simulink model "clearing_faulted_segment_travelling_Wave"  (R2018a)
settings: Solver=ode23t  StartTime=0.0  StopTime=2  MaxStep=1e-3  RelTol=1e-3
values from neighbouring files (symbols this model uses):
  AC_lim = [1.5 -1.5]    [MT_HVDC_initialize.m]
  C_pm = 10.48e-3    (= 0.01048)    [MT_HVDC_initialize.m]
  ccsc_lim = [1.0 -1.0]    [MT_HVDC_initialize.m]
  DC_lim = [1.05 -1.05]    [MT_HVDC_initialize.m]
  f = 50    [MT_HVDC_initialize.m]
  Fc = 50    [MT_HVDC_initialize.m]
  Fn_filter = 1000    [MT_HVDC_initialize.m]
  Ireg_lim_i = [1.5, -1.5]    [MT_HVDC_initialize.m]
  Ireg_lim_r = [1.5, -1.5]    [MT_HVDC_initialize.m]
  Ki_ACreg_i = 260    [MT_HVDC_initialize.m]
  Ki_ccsc = 5    [MT_HVDC_initialize.m]
  Ki_DCreg_r = 150    [MT_HVDC_initialize.m]
  Ki_Ireg_i = 200    [MT_HVDC_initialize.m]
  Ki_Ireg_r = 100    [MT_HVDC_initialize.m]
  Ki_R_inv = 150000    [MT_HVDC_initialize.m]
  Ki_R_rec = 5000    [MT_HVDC_initialize.m]
  Kp_ACreg_i = 2    [MT_HVDC_initialize.m]
  Kp_ccsc = 1    [MT_HVDC_initialize.m]
  Kp_DCreg_r = 8    [MT_HVDC_initialize.m]
  Kp_Ireg_i = 2    [MT_HVDC_initialize.m]
  Kp_Ireg_r = 2    [MT_HVDC_initialize.m]
  Kp_R_inv = 0.001    [MT_HVDC_initialize.m]
  Kp_R_rec = 0.001    [MT_HVDC_initialize.m]
  L1_pu = 0.109    [MT_HVDC_initialize.m]
  L2_pu = 0.0824    [MT_HVDC_initialize.m]
  L_arm = L_arm_pu*Z_base66/w    [MT_HVDC_initialize.m]
  L_arm_pu = 0.15    [MT_HVDC_initialize.m]
  L_int = X_int/w    [MT_HVDC_initialize.m]
  n = 50    [MT_HVDC_initialize.m]
  n2 = 50    [MT_HVDC_initialize.m]
  P_nom = 220e6    (= 220000000)    [MT_HVDC_initialize.m]
  R1_pu = 0.00206    [MT_HVDC_initialize.m]
  R2_pu = 0.00206    [MT_HVDC_initialize.m]
  R_arm = 0.03    [MT_HVDC_initialize.m]
  R_arm_pu = R_arm/Z_base66    [MT_HVDC_initialize.m]
  R_int = sqrt((z_int_400^2)/(1+xr_ratio^2))    [MT_HVDC_initialize.m]
  Rg_T1 = 40    [MT_HVDC_initialize.m]
  S1_nom = P_nom    (= 220000000)    [MT_HVDC_initialize.m]
  S2_nom = P_nom    (= 220000000)    [MT_HVDC_initialize.m]
  T_fault = 1.4    [MT_HVDC_initialize.m]
  Ts_Control = 40e-6    (= 4e-05)    [MT_HVDC_initialize.m]
  Ts_Power = 20e-6    (= 2e-05)    [MT_HVDC_initialize.m]
  V1_prim = V_prim    (= 400000)    [MT_HVDC_initialize.m]
  V1_sec = V_grid    (= 66000)    [MT_HVDC_initialize.m]
  V2_prim = V_grid    (= 66000)    [MT_HVDC_initialize.m]
  V2_sec = 18e3    (= 18000)    [MT_HVDC_initialize.m]
  V_ac_ref = 1.035    [MT_HVDC_initialize.m]
  V_grid = 66e3    (= 66000)    [MT_HVDC_initialize.m]
  V_prim = 400e3    (= 400000)    [MT_HVDC_initialize.m]
  Vc_pm_r = 0*Vdc_nom/n    (= 0)    [MT_HVDC_initialize.m]
  Vdc_nom = 135e3    (= 135000)    [MT_HVDC_initialize.m]
  w = 2*pi*f    (= 314.159265359)    [MT_HVDC_initialize.m]
  z0z1 = 0.8    [MT_HVDC_initialize.m]
  Zeta_filter = 1    [MT_HVDC_initialize.m]
undefined symbols (not defined in the file or in its folder): D1, Delta, DiscIntNeverNeededParam
libraries: powerlib x417, powerlib_meascontrol x130, simulink x84, powerlib_extras x8, simulink_extras x5
(part 14 of 17)

== system clearing_faulted_segment_travelling_Wave/MMC Converter2/Half-Bridge MMC Ap2/HalfBridgeMMC_Agt_Discrete ==
  N : Inport  PortDimensions=2
  Current Measurement1 : powerlib/Measurements/Current Measurement  PhasorSimulation=off  OutputType=Complex  PSBequivalent=0
      settings: SourceProductName=Simscape Electrical
  Current Measurement2 : powerlib/Measurements/Current Measurement  PhasorSimulation=off  OutputType=Complex  PSBequivalent=0
      settings: SourceProductName=Simscape Electrical
  Demux : Demux  Outputs=2
  Discrete-Time Integrator : DiscreteIntegrator  IntegratorMethod=Integration: Trapezoidal  gainval=1  InitialCondition=Vc_Initial  SampleTime=Ts  UpperSaturationLimit=5000  LowerSaturationLimit=500  ICPrevOutput=DiscIntNeverNeededParam  ICPrevScaledInput=DiscIntNeverNeededParam
  Dp : powerlib/Power Electronics/Diode  Ron=Ron_Diode  Lon=0  Vf=Vf_Diode  IC=0  UseSnubber=off  Rs=Rs_Diode  Cs=Cs_Diode  Measurements=off
      settings: SourceProductName=Simscape Electrical
  Dp2 : powerlib/Power Electronics/Diode  Ron=Ron_Diode  Lon=0  Vf=Vf_Diode  IC=0  UseSnubber=off  Rs=Rs_Diode  Cs=Cs_Diode  Measurements=off
      settings: SourceProductName=Simscape Electrical
  Gain : Gain  Gain=1/(C*n)
  Gain2 : Gain  Gain=2
  Mux : Mux  Inputs=2
  Product1 : Product
  Product2 : Product
  Saturation1 : Saturate  UpperLimit=n  LowerLimit=0
  Sum1 : Sum  Inputs=1  SaturateOnIntegerOverflow=on  InputSameDT=on  OutDataTypeStr=Inherit: Same as first input
  Sum2 : Sum  Inputs=+-  SaturateOnIntegerOverflow=on  InputSameDT=on  OutDataTypeStr=Inherit: Same as first input
  Unit Delay1 : UnitDelay  SampleTime=Ts
  Unit Delay3 : UnitDelay  InitialCondition=Vc_Initial  SampleTime=Ts
  Unit Delay4 : UnitDelay  InitialCondition=Vc_Initial  SampleTime=Ts
  Vp : powerlib/Electrical Sources/Controlled Voltage Source  Initialize=off  Source_Type=AC  Amplitude=0  Phase=0  Frequency=0  Measurements=None
      settings: SourceProductName=Simscape Electrical
  Vp1 : powerlib/Electrical Sources/Controlled Voltage Source  Initialize=off  Source_Type=AC  Amplitude=0  Phase=0  Frequency=0  Measurements=None
      settings: SourceProductName=Simscape Electrical
  1 : PMIOPort  Side=Left
  2 : PMIOPort  Port=2  Side=Left
  Vc : Outport
  wires:
  Sum1/1 -> Gain/1
  Sum2/1 -> Vc/1, Product2/2
  Product1/1 -> Sum1/1
  Saturation1/1 -> Product2/1, Product1/1
  Unit Delay1/1 -> Product1/2
  [Icap] -> Mux/2
  [Vbl] -> Vp1/1
  Current Measurement2/1 -> [Icap]
  Current Measurement1/1 -> [Imod]
  [Vin] -> Vp/1
  Demux/2 -> [Vbl]
  Demux/1 -> [Vin]
  Product2/1 -> Demux/1
  Mux/1 -> Unit Delay1/1
  Discrete-Time Integrator/1 -> Unit Delay4/1
  Gain/1 -> Discrete-Time Integrator/1
  Gain2/1 -> Sum2/1
  Unit Delay4/1 -> Gain2/1, Unit Delay3/1
  Unit Delay3/1 -> Sum2/2
  [Imod] -> Mux/1
  N/1 -> Saturation1/1
  connections:
  Dp2/LConn1 -- 2/RConn1 -- Vp1/LConn1
  Vp1/RConn1 -- Current Measurement2/RConn1
  Current Measurement2/LConn1 -- Dp/RConn1
  Dp2/RConn1 -- Dp/LConn1 -- Current Measurement1/RConn1
  Vp/LConn1 -- Current Measurement1/LConn1
  1/RConn1 -- Vp/RConn1

== system clearing_faulted_segment_travelling_Wave/MMC Converter2/Half-Bridge MMC Ap3/HalfBridgeMMC_Agt_Discrete ==
  N : Inport  PortDimensions=2
  Current Measurement1 : powerlib/Measurements/Current Measurement  PhasorSimulation=off  OutputType=Complex  PSBequivalent=0
      settings: SourceProductName=Simscape Electrical
  Current Measurement2 : powerlib/Measurements/Current Measurement  PhasorSimulation=off  OutputType=Complex  PSBequivalent=0
      settings: SourceProductName=Simscape Electrical
  Demux : Demux  Outputs=2
  Discrete-Time Integrator : DiscreteIntegrator  IntegratorMethod=Integration: Trapezoidal  gainval=1  InitialCondition=Vc_Initial  SampleTime=Ts  UpperSaturationLimit=5000  LowerSaturationLimit=500  ICPrevOutput=DiscIntNeverNeededParam  ICPrevScaledInput=DiscIntNeverNeededParam
  Dp : powerlib/Power Electronics/Diode  Ron=Ron_Diode  Lon=0  Vf=Vf_Diode  IC=0  UseSnubber=off  Rs=Rs_Diode  Cs=Cs_Diode  Measurements=off
      settings: SourceProductName=Simscape Electrical
  Dp2 : powerlib/Power Electronics/Diode  Ron=Ron_Diode  Lon=0  Vf=Vf_Diode  IC=0  UseSnubber=off  Rs=Rs_Diode  Cs=Cs_Diode  Measurements=off
      settings: SourceProductName=Simscape Electrical
  Gain : Gain  Gain=1/(C*n)
  Gain2 : Gain  Gain=2
  Mux : Mux  Inputs=2
  Product1 : Product
  Product2 : Product
  Saturation1 : Saturate  UpperLimit=n  LowerLimit=0
  Sum1 : Sum  Inputs=1  SaturateOnIntegerOverflow=on  InputSameDT=on  OutDataTypeStr=Inherit: Same as first input
  Sum2 : Sum  Inputs=+-  SaturateOnIntegerOverflow=on  InputSameDT=on  OutDataTypeStr=Inherit: Same as first input
  Unit Delay1 : UnitDelay  SampleTime=Ts
  Unit Delay3 : UnitDelay  InitialCondition=Vc_Initial  SampleTime=Ts
  Unit Delay4 : UnitDelay  InitialCondition=Vc_Initial  SampleTime=Ts
  Vp : powerlib/Electrical Sources/Controlled Voltage Source  Initialize=off  Source_Type=AC  Amplitude=0  Phase=0  Frequency=0  Measurements=None
      settings: SourceProductName=Simscape Electrical
  Vp1 : powerlib/Electrical Sources/Controlled Voltage Source  Initialize=off  Source_Type=AC  Amplitude=0  Phase=0  Frequency=0  Measurements=None
      settings: SourceProductName=Simscape Electrical
  1 : PMIOPort  Side=Left
  2 : PMIOPort  Port=2  Side=Left
  Vc : Outport
  wires:
  Sum1/1 -> Gain/1
  Sum2/1 -> Vc/1, Product2/2
  Product1/1 -> Sum1/1
  Saturation1/1 -> Product2/1, Product1/1
  Unit Delay1/1 -> Product1/2
  [Icap] -> Mux/2
  [Vbl] -> Vp1/1
  Current Measurement2/1 -> [Icap]
  Current Measurement1/1 -> [Imod]
  [Vin] -> Vp/1
  Demux/2 -> [Vbl]
  Demux/1 -> [Vin]
  Product2/1 -> Demux/1
  Mux/1 -> Unit Delay1/1
  Discrete-Time Integrator/1 -> Unit Delay4/1
  Gain/1 -> Discrete-Time Integrator/1
  Gain2/1 -> Sum2/1
  Unit Delay4/1 -> Gain2/1, Unit Delay3/1
  Unit Delay3/1 -> Sum2/2
  [Imod] -> Mux/1
  N/1 -> Saturation1/1
  connections:
  Dp2/LConn1 -- 2/RConn1 -- Vp1/LConn1
  Vp1/RConn1 -- Current Measurement2/RConn1
  Current Measurement2/LConn1 -- Dp/RConn1
  Dp2/RConn1 -- Dp/LConn1 -- Current Measurement1/RConn1
  Vp/LConn1 -- Current Measurement1/LConn1
  1/RConn1 -- Vp/RConn1

== system clearing_faulted_segment_travelling_Wave/MMC Converter2/Half-Bridge MMC Ap4/HalfBridgeMMC_Agt_Discrete ==
  N : Inport  PortDimensions=2
  Current Measurement1 : powerlib/Measurements/Current Measurement  PhasorSimulation=off  OutputType=Complex  PSBequivalent=0
      settings: SourceProductName=Simscape Electrical
  Current Measurement2 : powerlib/Measurements/Current Measurement  PhasorSimulation=off  OutputType=Complex  PSBequivalent=0
      settings: SourceProductName=Simscape Electrical
  Demux : Demux  Outputs=2
  Discrete-Time Integrator : DiscreteIntegrator  IntegratorMethod=Integration: Trapezoidal  gainval=1  InitialCondition=Vc_Initial  SampleTime=Ts  UpperSaturationLimit=5000  LowerSaturationLimit=500  ICPrevOutput=DiscIntNeverNeededParam  ICPrevScaledInput=DiscIntNeverNeededParam
  Dp : powerlib/Power Electronics/Diode  Ron=Ron_Diode  Lon=0  Vf=Vf_Diode  IC=0  UseSnubber=off  Rs=Rs_Diode  Cs=Cs_Diode  Measurements=off
      settings: SourceProductName=Simscape Electrical
  Dp2 : powerlib/Power Electronics/Diode  Ron=Ron_Diode  Lon=0  Vf=Vf_Diode  IC=0  UseSnubber=off  Rs=Rs_Diode  Cs=Cs_Diode  Measurements=off
      settings: SourceProductName=Simscape Electrical
  Gain : Gain  Gain=1/(C*n)
  Gain2 : Gain  Gain=2
  Mux : Mux  Inputs=2
  Product1 : Product
  Product2 : Product
  Saturation1 : Saturate  UpperLimit=n  LowerLimit=0
  Sum1 : Sum  Inputs=1  SaturateOnIntegerOverflow=on  InputSameDT=on  OutDataTypeStr=Inherit: Same as first input
  Sum2 : Sum  Inputs=+-  SaturateOnIntegerOverflow=on  InputSameDT=on  OutDataTypeStr=Inherit: Same as first input
  Unit Delay1 : UnitDelay  SampleTime=Ts
  Unit Delay3 : UnitDelay  InitialCondition=Vc_Initial  SampleTime=Ts
  Unit Delay4 : UnitDelay  InitialCondition=Vc_Initial  SampleTime=Ts
  Vp : powerlib/Electrical Sources/Controlled Voltage Source  Initialize=off  Source_Type=AC  Amplitude=0  Phase=0  Frequency=0  Measurements=None
      settings: SourceProductName=Simscape Electrical
  Vp1 : powerlib/Electrical Sources/Controlled Voltage Source  Initialize=off  Source_Type=AC  Amplitude=0  Phase=0  Frequency=0  Measurements=None
      settings: SourceProductName=Simscape Electrical
  1 : PMIOPort  Side=Left
  2 : PMIOPort  Port=2  Side=Left
  Vc : Outport
  wires:
  N/1 -> Saturation1/1
  [Imod] -> Mux/1
  Unit Delay3/1 -> Sum2/2
  Unit Delay4/1 -> Unit Delay3/1, Gain2/1
  Gain2/1 -> Sum2/1
  Gain/1 -> Discrete-Time Integrator/1
  Discrete-Time Integrator/1 -> Unit Delay4/1
  Mux/1 -> Unit Delay1/1
  Product2/1 -> Demux/1
  Demux/1 -> [Vin]
  Demux/2 -> [Vbl]
  [Vin] -> Vp/1
  Current Measurement1/1 -> [Imod]
  Current Measurement2/1 -> [Icap]
  [Vbl] -> Vp1/1
  [Icap] -> Mux/2
  Unit Delay1/1 -> Product1/2
  Saturation1/1 -> Product1/1, Product2/1
  Product1/1 -> Sum1/1
  Sum2/1 -> Product2/2, Vc/1
  Sum1/1 -> Gain/1
  connections:
  1/RConn1 -- Vp/RConn1
  Vp/LConn1 -- Current Measurement1/LConn1
  Current Measurement1/RConn1 -- Dp/LConn1 -- Dp2/RConn1
  Current Measurement2/LConn1 -- Dp/RConn1
  Vp1/RConn1 -- Current Measurement2/RConn1
  Vp1/LConn1 -- 2/RConn1 -- Dp2/LConn1

== system clearing_faulted_segment_travelling_Wave/MMC Converter2/Half-Bridge MMC Ap5/HalfBridgeMMC_Agt_Discrete ==
  N : Inport  PortDimensions=2
  Current Measurement1 : powerlib/Measurements/Current Measurement  PhasorSimulation=off  OutputType=Complex  PSBequivalent=0
      settings: SourceProductName=Simscape Electrical
  Current Measurement2 : powerlib/Measurements/Current Measurement  PhasorSimulation=off  OutputType=Complex  PSBequivalent=0
      settings: SourceProductName=Simscape Electrical
  Demux : Demux  Outputs=2
  Discrete-Time Integrator : DiscreteIntegrator  IntegratorMethod=Integration: Trapezoidal  gainval=1  InitialCondition=Vc_Initial  SampleTime=Ts  UpperSaturationLimit=5000  LowerSaturationLimit=500  ICPrevOutput=DiscIntNeverNeededParam  ICPrevScaledInput=DiscIntNeverNeededParam
  Dp : powerlib/Power Electronics/Diode  Ron=Ron_Diode  Lon=0  Vf=Vf_Diode  IC=0  UseSnubber=off  Rs=Rs_Diode  Cs=Cs_Diode  Measurements=off
      settings: SourceProductName=Simscape Electrical
  Dp2 : powerlib/Power Electronics/Diode  Ron=Ron_Diode  Lon=0  Vf=Vf_Diode  IC=0  UseSnubber=off  Rs=Rs_Diode  Cs=Cs_Diode  Measurements=off
      settings: SourceProductName=Simscape Electrical
  Gain : Gain  Gain=1/(C*n)
  Gain2 : Gain  Gain=2
  Mux : Mux  Inputs=2
  Product1 : Product
  Product2 : Product
  Saturation1 : Saturate  UpperLimit=n  LowerLimit=0
  Sum1 : Sum  Inputs=1  SaturateOnIntegerOverflow=on  InputSameDT=on  OutDataTypeStr=Inherit: Same as first input
  Sum2 : Sum  Inputs=+-  SaturateOnIntegerOverflow=on  InputSameDT=on  OutDataTypeStr=Inherit: Same as first input
  Unit Delay1 : UnitDelay  SampleTime=Ts
  Unit Delay3 : UnitDelay  InitialCondition=Vc_Initial  SampleTime=Ts
  Unit Delay4 : UnitDelay  InitialCondition=Vc_Initial  SampleTime=Ts
  Vp : powerlib/Electrical Sources/Controlled Voltage Source  Initialize=off  Source_Type=AC  Amplitude=0  Phase=0  Frequency=0  Measurements=None
      settings: SourceProductName=Simscape Electrical
  Vp1 : powerlib/Electrical Sources/Controlled Voltage Source  Initialize=off  Source_Type=AC  Amplitude=0  Phase=0  Frequency=0  Measurements=None
      settings: SourceProductName=Simscape Electrical
  1 : PMIOPort  Side=Left
  2 : PMIOPort  Port=2  Side=Left
  Vc : Outport
  wires:
  Sum1/1 -> Gain/1
  Sum2/1 -> Vc/1, Product2/2
  Product1/1 -> Sum1/1
  Saturation1/1 -> Product2/1, Product1/1
  Unit Delay1/1 -> Product1/2
  [Icap] -> Mux/2
  [Vbl] -> Vp1/1
  Current Measurement2/1 -> [Icap]
  Current Measurement1/1 -> [Imod]
  [Vin] -> Vp/1
  Demux/2 -> [Vbl]
  Demux/1 -> [Vin]
  Product2/1 -> Demux/1
  Mux/1 -> Unit Delay1/1
  Discrete-Time Integrator/1 -> Unit Delay4/1
  Gain/1 -> Discrete-Time Integrator/1
  Gain2/1 -> Sum2/1
  Unit Delay4/1 -> Gain2/1, Unit Delay3/1
  Unit Delay3/1 -> Sum2/2
  [Imod] -> Mux/1
  N/1 -> Saturation1/1
  connections:
  Dp2/LConn1 -- 2/RConn1 -- Vp1/LConn1
  Vp1/RConn1 -- Current Measurement2/RConn1
  Current Measurement2/LConn1 -- Dp/RConn1
  Dp2/RConn1 -- Dp/LConn1 -- Current Measurement1/RConn1
  Vp/LConn1 -- Current Measurement1/LConn1
  1/RConn1 -- Vp/RConn1

== system clearing_faulted_segment_travelling_Wave/MMC Converter3/Half-Bridge MMC Ap/HalfBridgeMMC_Agt_Discrete ==
  N : Inport  PortDimensions=2
  Current Measurement1 : powerlib/Measurements/Current Measurement  PhasorSimulation=off  OutputType=Complex  PSBequivalent=0
      settings: SourceProductName=Simscape Electrical
  Current Measurement2 : powerlib/Measurements/Current Measurement  PhasorSimulation=off  OutputType=Complex  PSBequivalent=0
      settings: SourceProductName=Simscape Electrical
  Demux : Demux  Outputs=2
  Discrete-Time Integrator : DiscreteIntegrator  IntegratorMethod=Integration: Trapezoidal  gainval=1  InitialCondition=Vc_Initial  SampleTime=Ts  UpperSaturationLimit=5000  LowerSaturationLimit=500  ICPrevOutput=DiscIntNeverNeededParam  ICPrevScaledInput=DiscIntNeverNeededParam
  Dp : powerlib/Power Electronics/Diode  Ron=Ron_Diode  Lon=0  Vf=Vf_Diode  IC=0  UseSnubber=off  Rs=Rs_Diode  Cs=Cs_Diode  Measurements=off
      settings: SourceProductName=Simscape Electrical
  Dp2 : powerlib/Power Electronics/Diode  Ron=Ron_Diode  Lon=0  Vf=Vf_Diode  IC=0  UseSnubber=off  Rs=Rs_Diode  Cs=Cs_Diode  Measurements=off
      settings: SourceProductName=Simscape Electrical
  Gain : Gain  Gain=1/(C*n)
  Gain2 : Gain  Gain=2
  Mux : Mux  Inputs=2
  Product1 : Product
  Product2 : Product
  Saturation1 : Saturate  UpperLimit=n  LowerLimit=0
  Sum1 : Sum  Inputs=1  SaturateOnIntegerOverflow=on  InputSameDT=on  OutDataTypeStr=Inherit: Same as first input
  Sum2 : Sum  Inputs=+-  SaturateOnIntegerOverflow=on  InputSameDT=on  OutDataTypeStr=Inherit: Same as first input
  Unit Delay1 : UnitDelay  SampleTime=Ts
  Unit Delay3 : UnitDelay  InitialCondition=Vc_Initial  SampleTime=Ts
  Unit Delay4 : UnitDelay  InitialCondition=Vc_Initial  SampleTime=Ts
  Vp : powerlib/Electrical Sources/Controlled Voltage Source  Initialize=off  Source_Type=AC  Amplitude=0  Phase=0  Frequency=0  Measurements=None
      settings: SourceProductName=Simscape Electrical
  Vp1 : powerlib/Electrical Sources/Controlled Voltage Source  Initialize=off  Source_Type=AC  Amplitude=0  Phase=0  Frequency=0  Measurements=None
      settings: SourceProductName=Simscape Electrical
  1 : PMIOPort  Side=Left
  2 : PMIOPort  Port=2  Side=Left
  Vc : Outport
  wires:
  N/1 -> Saturation1/1
  [Imod] -> Mux/1
  Unit Delay3/1 -> Sum2/2
  Unit Delay4/1 -> Unit Delay3/1, Gain2/1
  Gain2/1 -> Sum2/1
  Gain/1 -> Discrete-Time Integrator/1
  Discrete-Time Integrator/1 -> Unit Delay4/1
  Mux/1 -> Unit Delay1/1
  Product2/1 -> Demux/1
  Demux/1 -> [Vin]
  Demux/2 -> [Vbl]
  [Vin] -> Vp/1
  Current Measurement1/1 -> [Imod]
  Current Measurement2/1 -> [Icap]
  [Vbl] -> Vp1/1
  [Icap] -> Mux/2
  Unit Delay1/1 -> Product1/2
  Saturation1/1 -> Product1/1, Product2/1
  Product1/1 -> Sum1/1
  Sum2/1 -> Product2/2, Vc/1
  Sum1/1 -> Gain/1
  connections:
  1/RConn1 -- Vp/RConn1
  Vp/LConn1 -- Current Measurement1/LConn1
  Current Measurement1/RConn1 -- Dp/LConn1 -- Dp2/RConn1
  Current Measurement2/LConn1 -- Dp/RConn1
  Vp1/RConn1 -- Current Measurement2/RConn1
  Vp1/LConn1 -- 2/RConn1 -- Dp2/LConn1

== system clearing_faulted_segment_travelling_Wave/MMC Converter3/Half-Bridge MMC Ap1/HalfBridgeMMC_Agt_Discrete ==
  N : Inport  PortDimensions=2
  Current Measurement1 : powerlib/Measurements/Current Measurement  PhasorSimulation=off  OutputType=Complex  PSBequivalent=0
      settings: SourceProductName=Simscape Electrical
  Current Measurement2 : powerlib/Measurements/Current Measurement  PhasorSimulation=off  OutputType=Complex  PSBequivalent=0
      settings: SourceProductName=Simscape Electrical
  Demux : Demux  Outputs=2
  Discrete-Time Integrator : DiscreteIntegrator  IntegratorMethod=Integration: Trapezoidal  gainval=1  InitialCondition=Vc_Initial  SampleTime=Ts  UpperSaturationLimit=5000  LowerSaturationLimit=500  ICPrevOutput=DiscIntNeverNeededParam  ICPrevScaledInput=DiscIntNeverNeededParam
  Dp : powerlib/Power Electronics/Diode  Ron=Ron_Diode  Lon=0  Vf=Vf_Diode  IC=0  UseSnubber=off  Rs=Rs_Diode  Cs=Cs_Diode  Measurements=off
      settings: SourceProductName=Simscape Electrical
  Dp2 : powerlib/Power Electronics/Diode  Ron=Ron_Diode  Lon=0  Vf=Vf_Diode  IC=0  UseSnubber=off  Rs=Rs_Diode  Cs=Cs_Diode  Measurements=off
      settings: SourceProductName=Simscape Electrical
  Gain : Gain  Gain=1/(C*n)
  Gain2 : Gain  Gain=2
  Mux : Mux  Inputs=2
  Product1 : Product
  Product2 : Product
  Saturation1 : Saturate  UpperLimit=n  LowerLimit=0
  Sum1 : Sum  Inputs=1  SaturateOnIntegerOverflow=on  InputSameDT=on  OutDataTypeStr=Inherit: Same as first input
  Sum2 : Sum  Inputs=+-  SaturateOnIntegerOverflow=on  InputSameDT=on  OutDataTypeStr=Inherit: Same as first input
  Unit Delay1 : UnitDelay  SampleTime=Ts
  Unit Delay3 : UnitDelay  InitialCondition=Vc_Initial  SampleTime=Ts
  Unit Delay4 : UnitDelay  InitialCondition=Vc_Initial  SampleTime=Ts
  Vp : powerlib/Electrical Sources/Controlled Voltage Source  Initialize=off  Source_Type=AC  Amplitude=0  Phase=0  Frequency=0  Measurements=None
      settings: SourceProductName=Simscape Electrical
  Vp1 : powerlib/Electrical Sources/Controlled Voltage Source  Initialize=off  Source_Type=AC  Amplitude=0  Phase=0  Frequency=0  Measurements=None
      settings: SourceProductName=Simscape Electrical
  1 : PMIOPort  Side=Left
  2 : PMIOPort  Port=2  Side=Left
  Vc : Outport
  wires:
  N/1 -> Saturation1/1
  [Imod] -> Mux/1
  Unit Delay3/1 -> Sum2/2
  Unit Delay4/1 -> Unit Delay3/1, Gain2/1
  Gain2/1 -> Sum2/1
  Gain/1 -> Discrete-Time Integrator/1
  Discrete-Time Integrator/1 -> Unit Delay4/1
  Mux/1 -> Unit Delay1/1
  Product2/1 -> Demux/1
  Demux/1 -> [Vin]
  Demux/2 -> [Vbl]
  [Vin] -> Vp/1
  Current Measurement1/1 -> [Imod]
  Current Measurement2/1 -> [Icap]
  [Vbl] -> Vp1/1
  [Icap] -> Mux/2
  Unit Delay1/1 -> Product1/2
  Saturation1/1 -> Product1/1, Product2/1
  Product1/1 -> Sum1/1
  Sum2/1 -> Product2/2, Vc/1
  Sum1/1 -> Gain/1
  connections:
  1/RConn1 -- Vp/RConn1
  Vp/LConn1 -- Current Measurement1/LConn1
  Current Measurement1/RConn1 -- Dp/LConn1 -- Dp2/RConn1
  Current Measurement2/LConn1 -- Dp/RConn1
  Vp1/RConn1 -- Current Measurement2/RConn1
  Vp1/LConn1 -- 2/RConn1 -- Dp2/LConn1

== system clearing_faulted_segment_travelling_Wave/MMC Converter3/Half-Bridge MMC Ap2/HalfBridgeMMC_Agt_Discrete ==
  N : Inport  PortDimensions=2
  Current Measurement1 : powerlib/Measurements/Current Measurement  PhasorSimulation=off  OutputType=Complex  PSBequivalent=0
      settings: SourceProductName=Simscape Electrical
  Current Measurement2 : powerlib/Measurements/Current Measurement  PhasorSimulation=off  OutputType=Complex  PSBequivalent=0
      settings: SourceProductName=Simscape Electrical
  Demux : Demux  Outputs=2
  Discrete-Time Integrator : DiscreteIntegrator  IntegratorMethod=Integration: Trapezoidal  gainval=1  InitialCondition=Vc_Initial  SampleTime=Ts  UpperSaturationLimit=5000  LowerSaturationLimit=500  ICPrevOutput=DiscIntNeverNeededParam  ICPrevScaledInput=DiscIntNeverNeededParam
  Dp : powerlib/Power Electronics/Diode  Ron=Ron_Diode  Lon=0  Vf=Vf_Diode  IC=0  UseSnubber=off  Rs=Rs_Diode  Cs=Cs_Diode  Measurements=off
      settings: SourceProductName=Simscape Electrical
  Dp2 : powerlib/Power Electronics/Diode  Ron=Ron_Diode  Lon=0  Vf=Vf_Diode  IC=0  UseSnubber=off  Rs=Rs_Diode  Cs=Cs_Diode  Measurements=off
      settings: SourceProductName=Simscape Electrical
  Gain : Gain  Gain=1/(C*n)
  Gain2 : Gain  Gain=2
  Mux : Mux  Inputs=2
  Product1 : Product
  Product2 : Product
  Saturation1 : Saturate  UpperLimit=n  LowerLimit=0
  Sum1 : Sum  Inputs=1  SaturateOnIntegerOverflow=on  InputSameDT=on  OutDataTypeStr=Inherit: Same as first input
  Sum2 : Sum  Inputs=+-  SaturateOnIntegerOverflow=on  InputSameDT=on  OutDataTypeStr=Inherit: Same as first input
  Unit Delay1 : UnitDelay  SampleTime=Ts
  Unit Delay3 : UnitDelay  InitialCondition=Vc_Initial  SampleTime=Ts
  Unit Delay4 : UnitDelay  InitialCondition=Vc_Initial  SampleTime=Ts
  Vp : powerlib/Electrical Sources/Controlled Voltage Source  Initialize=off  Source_Type=AC  Amplitude=0  Phase=0  Frequency=0  Measurements=None
      settings: SourceProductName=Simscape Electrical
  Vp1 : powerlib/Electrical Sources/Controlled Voltage Source  Initialize=off  Source_Type=AC  Amplitude=0  Phase=0  Frequency=0  Measurements=None
      settings: SourceProductName=Simscape Electrical
  1 : PMIOPort  Side=Left
  2 : PMIOPort  Port=2  Side=Left
  Vc : Outport
  wires:
  Sum1/1 -> Gain/1
  Sum2/1 -> Vc/1, Product2/2
  Product1/1 -> Sum1/1
  Saturation1/1 -> Product2/1, Product1/1
  Unit Delay1/1 -> Product1/2
  [Icap] -> Mux/2
  [Vbl] -> Vp1/1
  Current Measurement2/1 -> [Icap]
  Current Measurement1/1 -> [Imod]
  [Vin] -> Vp/1
  Demux/2 -> [Vbl]
  Demux/1 -> [Vin]
  Product2/1 -> Demux/1
  Mux/1 -> Unit Delay1/1
  Discrete-Time Integrator/1 -> Unit Delay4/1
  Gain/1 -> Discrete-Time Integrator/1
  Gain2/1 -> Sum2/1
  Unit Delay4/1 -> Gain2/1, Unit Delay3/1
  Unit Delay3/1 -> Sum2/2
  [Imod] -> Mux/1
  N/1 -> Saturation1/1
  connections:
  Dp2/LConn1 -- 2/RConn1 -- Vp1/LConn1
  Vp1/RConn1 -- Current Measurement2/RConn1
  Current Measurement2/LConn1 -- Dp/RConn1
  Dp2/RConn1 -- Dp/LConn1 -- Current Measurement1/RConn1
  Vp/LConn1 -- Current Measurement1/LConn1
  1/RConn1 -- Vp/RConn1

== system clearing_faulted_segment_travelling_Wave/MMC Converter3/Half-Bridge MMC Ap3/HalfBridgeMMC_Agt_Discrete ==
  N : Inport  PortDimensions=2
  Current Measurement1 : powerlib/Measurements/Current Measurement  PhasorSimulation=off  OutputType=Complex  PSBequivalent=0
      settings: SourceProductName=Simscape Electrical
  Current Measurement2 : powerlib/Measurements/Current Measurement  PhasorSimulation=off  OutputType=Complex  PSBequivalent=0
      settings: SourceProductName=Simscape Electrical
  Demux : Demux  Outputs=2
  Discrete-Time Integrator : DiscreteIntegrator  IntegratorMethod=Integration: Trapezoidal  gainval=1  InitialCondition=Vc_Initial  SampleTime=Ts  UpperSaturationLimit=5000  LowerSaturationLimit=500  ICPrevOutput=DiscIntNeverNeededParam  ICPrevScaledInput=DiscIntNeverNeededParam
  Dp : powerlib/Power Electronics/Diode  Ron=Ron_Diode  Lon=0  Vf=Vf_Diode  IC=0  UseSnubber=off  Rs=Rs_Diode  Cs=Cs_Diode  Measurements=off
      settings: SourceProductName=Simscape Electrical
  Dp2 : powerlib/Power Electronics/Diode  Ron=Ron_Diode  Lon=0  Vf=Vf_Diode  IC=0  UseSnubber=off  Rs=Rs_Diode  Cs=Cs_Diode  Measurements=off
      settings: SourceProductName=Simscape Electrical
  Gain : Gain  Gain=1/(C*n)
  Gain2 : Gain  Gain=2
  Mux : Mux  Inputs=2
  Product1 : Product
  Product2 : Product
  Saturation1 : Saturate  UpperLimit=n  LowerLimit=0
  Sum1 : Sum  Inputs=1  SaturateOnIntegerOverflow=on  InputSameDT=on  OutDataTypeStr=Inherit: Same as first input
  Sum2 : Sum  Inputs=+-  SaturateOnIntegerOverflow=on  InputSameDT=on  OutDataTypeStr=Inherit: Same as first input
  Unit Delay1 : UnitDelay  SampleTime=Ts
  Unit Delay3 : UnitDelay  InitialCondition=Vc_Initial  SampleTime=Ts
  Unit Delay4 : UnitDelay  InitialCondition=Vc_Initial  SampleTime=Ts
  Vp : powerlib/Electrical Sources/Controlled Voltage Source  Initialize=off  Source_Type=AC  Amplitude=0  Phase=0  Frequency=0  Measurements=None
      settings: SourceProductName=Simscape Electrical
  Vp1 : powerlib/Electrical Sources/Controlled Voltage Source  Initialize=off  Source_Type=AC  Amplitude=0  Phase=0  Frequency=0  Measurements=None
      settings: SourceProductName=Simscape Electrical
  1 : PMIOPort  Side=Left
  2 : PMIOPort  Port=2  Side=Left
  Vc : Outport
  wires:
  Sum1/1 -> Gain/1
  Sum2/1 -> Vc/1, Product2/2
  Product1/1 -> Sum1/1
  Saturation1/1 -> Product2/1, Product1/1
  Unit Delay1/1 -> Product1/2
  [Icap] -> Mux/2
  [Vbl] -> Vp1/1
  Current Measurement2/1 -> [Icap]
  Current Measurement1/1 -> [Imod]
  [Vin] -> Vp/1
  Demux/2 -> [Vbl]
  Demux/1 -> [Vin]
  Product2/1 -> Demux/1
  Mux/1 -> Unit Delay1/1
  Discrete-Time Integrator/1 -> Unit Delay4/1
  Gain/1 -> Discrete-Time Integrator/1
  Gain2/1 -> Sum2/1
  Unit Delay4/1 -> Gain2/1, Unit Delay3/1
  Unit Delay3/1 -> Sum2/2
  [Imod] -> Mux/1
  N/1 -> Saturation1/1
  connections:
  Dp2/LConn1 -- 2/RConn1 -- Vp1/LConn1
  Vp1/RConn1 -- Current Measurement2/RConn1
  Current Measurement2/LConn1 -- Dp/RConn1
  Dp2/RConn1 -- Dp/LConn1 -- Current Measurement1/RConn1
  Vp/LConn1 -- Current Measurement1/LConn1
  1/RConn1 -- Vp/RConn1

== system clearing_faulted_segment_travelling_Wave/MMC Converter3/Half-Bridge MMC Ap4/HalfBridgeMMC_Agt_Discrete ==
  N : Inport  PortDimensions=2
  Current Measurement1 : powerlib/Measurements/Current Measurement  PhasorSimulation=off  OutputType=Complex  PSBequivalent=0
      settings: SourceProductName=Simscape Electrical
  Current Measurement2 : powerlib/Measurements/Current Measurement  PhasorSimulation=off  OutputType=Complex  PSBequivalent=0
      settings: SourceProductName=Simscape Electrical
  Demux : Demux  Outputs=2
  Discrete-Time Integrator : DiscreteIntegrator  IntegratorMethod=Integration: Trapezoidal  gainval=1  InitialCondition=Vc_Initial  SampleTime=Ts  UpperSaturationLimit=5000  LowerSaturationLimit=500  ICPrevOutput=DiscIntNeverNeededParam  ICPrevScaledInput=DiscIntNeverNeededParam
  Dp : powerlib/Power Electronics/Diode  Ron=Ron_Diode  Lon=0  Vf=Vf_Diode  IC=0  UseSnubber=off  Rs=Rs_Diode  Cs=Cs_Diode  Measurements=off
      settings: SourceProductName=Simscape Electrical
  Dp2 : powerlib/Power Electronics/Diode  Ron=Ron_Diode  Lon=0  Vf=Vf_Diode  IC=0  UseSnubber=off  Rs=Rs_Diode  Cs=Cs_Diode  Measurements=off
      settings: SourceProductName=Simscape Electrical
  Gain : Gain  Gain=1/(C*n)
  Gain2 : Gain  Gain=2
  Mux : Mux  Inputs=2
  Product1 : Product
  Product2 : Product
  Saturation1 : Saturate  UpperLimit=n  LowerLimit=0
  Sum1 : Sum  Inputs=1  SaturateOnIntegerOverflow=on  InputSameDT=on  OutDataTypeStr=Inherit: Same as first input
  Sum2 : Sum  Inputs=+-  SaturateOnIntegerOverflow=on  InputSameDT=on  OutDataTypeStr=Inherit: Same as first input
  Unit Delay1 : UnitDelay  SampleTime=Ts
  Unit Delay3 : UnitDelay  InitialCondition=Vc_Initial  SampleTime=Ts
  Unit Delay4 : UnitDelay  InitialCondition=Vc_Initial  SampleTime=Ts
  Vp : powerlib/Electrical Sources/Controlled Voltage Source  Initialize=off  Source_Type=AC  Amplitude=0  Phase=0  Frequency=0  Measurements=None
      settings: SourceProductName=Simscape Electrical
  Vp1 : powerlib/Electrical Sources/Controlled Voltage Source  Initialize=off  Source_Type=AC  Amplitude=0  Phase=0  Frequency=0  Measurements=None
      settings: SourceProductName=Simscape Electrical
  1 : PMIOPort  Side=Left
  2 : PMIOPort  Port=2  Side=Left
  Vc : Outport
  wires:
  N/1 -> Saturation1/1
  [Imod] -> Mux/1
  Unit Delay3/1 -> Sum2/2
  Unit Delay4/1 -> Unit Delay3/1, Gain2/1
  Gain2/1 -> Sum2/1
  Gain/1 -> Discrete-Time Integrator/1
  Discrete-Time Integrator/1 -> Unit Delay4/1
  Mux/1 -> Unit Delay1/1
  Product2/1 -> Demux/1
  Demux/1 -> [Vin]
  Demux/2 -> [Vbl]
  [Vin] -> Vp/1
  Current Measurement1/1 -> [Imod]
  Current Measurement2/1 -> [Icap]
  [Vbl] -> Vp1/1
  [Icap] -> Mux/2
  Unit Delay1/1 -> Product1/2
  Saturation1/1 -> Product1/1, Product2/1
  Product1/1 -> Sum1/1
  Sum2/1 -> Product2/2, Vc/1
  Sum1/1 -> Gain/1
  connections:
  1/RConn1 -- Vp/RConn1
  Vp/LConn1 -- Current Measurement1/LConn1
  Current Measurement1/RConn1 -- Dp/LConn1 -- Dp2/RConn1
  Current Measurement2/LConn1 -- Dp/RConn1
  Vp1/RConn1 -- Current Measurement2/RConn1
  Vp1/LConn1 -- 2/RConn1 -- Dp2/LConn1

== system clearing_faulted_segment_travelling_Wave/MMC Converter3/Half-Bridge MMC Ap5/HalfBridgeMMC_Agt_Discrete ==
  N : Inport  PortDimensions=2
  Current Measurement1 : powerlib/Measurements/Current Measurement  PhasorSimulation=off  OutputType=Complex  PSBequivalent=0
      settings: SourceProductName=Simscape Electrical
  Current Measurement2 : powerlib/Measurements/Current Measurement  PhasorSimulation=off  OutputType=Complex  PSBequivalent=0
      settings: SourceProductName=Simscape Electrical
  Demux : Demux  Outputs=2
  Discrete-Time Integrator : DiscreteIntegrator  IntegratorMethod=Integration: Trapezoidal  gainval=1  InitialCondition=Vc_Initial  SampleTime=Ts  UpperSaturationLimit=5000  LowerSaturationLimit=500  ICPrevOutput=DiscIntNeverNeededParam  ICPrevScaledInput=DiscIntNeverNeededParam
  Dp : powerlib/Power Electronics/Diode  Ron=Ron_Diode  Lon=0  Vf=Vf_Diode  IC=0  UseSnubber=off  Rs=Rs_Diode  Cs=Cs_Diode  Measurements=off
      settings: SourceProductName=Simscape Electrical
  Dp2 : powerlib/Power Electronics/Diode  Ron=Ron_Diode  Lon=0  Vf=Vf_Diode  IC=0  UseSnubber=off  Rs=Rs_Diode  Cs=Cs_Diode  Measurements=off
      settings: SourceProductName=Simscape Electrical
  Gain : Gain  Gain=1/(C*n)
  Gain2 : Gain  Gain=2
  Mux : Mux  Inputs=2
  Product1 : Product
  Product2 : Product
  Saturation1 : Saturate  UpperLimit=n  LowerLimit=0
  Sum1 : Sum  Inputs=1  SaturateOnIntegerOverflow=on  InputSameDT=on  OutDataTypeStr=Inherit: Same as first input
  Sum2 : Sum  Inputs=+-  SaturateOnIntegerOverflow=on  InputSameDT=on  OutDataTypeStr=Inherit: Same as first input
  Unit Delay1 : UnitDelay  SampleTime=Ts
  Unit Delay3 : UnitDelay  InitialCondition=Vc_Initial  SampleTime=Ts
  Unit Delay4 : UnitDelay  InitialCondition=Vc_Initial  SampleTime=Ts
  Vp : powerlib/Electrical Sources/Controlled Voltage Source  Initialize=off  Source_Type=AC  Amplitude=0  Phase=0  Frequency=0  Measurements=None
      settings: SourceProductName=Simscape Electrical
  Vp1 : powerlib/Electrical Sources/Controlled Voltage Source  Initialize=off  Source_Type=AC  Amplitude=0  Phase=0  Frequency=0  Measurements=None
      settings: SourceProductName=Simscape Electrical
  1 : PMIOPort  Side=Left
  2 : PMIOPort  Port=2  Side=Left
  Vc : Outport
  wires:
  Sum1/1 -> Gain/1
  Sum2/1 -> Vc/1, Product2/2
  Product1/1 -> Sum1/1
  Saturation1/1 -> Product2/1, Product1/1
  Unit Delay1/1 -> Product1/2
  [Icap] -> Mux/2
  [Vbl] -> Vp1/1
  Current Measurement2/1 -> [Icap]
  Current Measurement1/1 -> [Imod]
  [Vin] -> Vp/1
  Demux/2 -> [Vbl]
  Demux/1 -> [Vin]
  Product2/1 -> Demux/1
  Mux/1 -> Unit Delay1/1
  Discrete-Time Integrator/1 -> Unit Delay4/1
  Gain/1 -> Discrete-Time Integrator/1
  Gain2/1 -> Sum2/1
  Unit Delay4/1 -> Gain2/1, Unit Delay3/1
  Unit Delay3/1 -> Sum2/2
  [Imod] -> Mux/1
  N/1 -> Saturation1/1
  connections:
  Dp2/LConn1 -- 2/RConn1 -- Vp1/LConn1
  Vp1/RConn1 -- Current Measurement2/RConn1
  Current Measurement2/LConn1 -- Dp/RConn1
  Dp2/RConn1 -- Dp/LConn1 -- Current Measurement1/RConn1
  Vp/LConn1 -- Current Measurement1/LConn1
  1/RConn1 -- Vp/RConn1

== system clearing_faulted_segment_travelling_Wave/MMC Converter4/Half-Bridge MMC Ap/HalfBridgeMMC_Agt_Discrete ==
  N : Inport  PortDimensions=2
  Current Measurement1 : powerlib/Measurements/Current Measurement  PhasorSimulation=off  OutputType=Complex  PSBequivalent=0
      settings: SourceProductName=Simscape Electrical
  Current Measurement2 : powerlib/Measurements/Current Measurement  PhasorSimulation=off  OutputType=Complex  PSBequivalent=0
      settings: SourceProductName=Simscape Electrical
  Demux : Demux  Outputs=2
  Discrete-Time Integrator : DiscreteIntegrator  IntegratorMethod=Integration: Trapezoidal  gainval=1  InitialCondition=Vc_Initial  SampleTime=Ts  UpperSaturationLimit=5000  LowerSaturationLimit=500  ICPrevOutput=DiscIntNeverNeededParam  ICPrevScaledInput=DiscIntNeverNeededParam
  Dp : powerlib/Power Electronics/Diode  Ron=Ron_Diode  Lon=0  Vf=Vf_Diode  IC=0  UseSnubber=off  Rs=Rs_Diode  Cs=Cs_Diode  Measurements=off
      settings: SourceProductName=Simscape Electrical
  Dp2 : powerlib/Power Electronics/Diode  Ron=Ron_Diode  Lon=0  Vf=Vf_Diode  IC=0  UseSnubber=off  Rs=Rs_Diode  Cs=Cs_Diode  Measurements=off
      settings: SourceProductName=Simscape Electrical
  Gain : Gain  Gain=1/(C*n)
  Gain2 : Gain  Gain=2
  Mux : Mux  Inputs=2
  Product1 : Product
  Product2 : Product
  Saturation1 : Saturate  UpperLimit=n  LowerLimit=0
  Sum1 : Sum  Inputs=1  SaturateOnIntegerOverflow=on  InputSameDT=on  OutDataTypeStr=Inherit: Same as first input
  Sum2 : Sum  Inputs=+-  SaturateOnIntegerOverflow=on  InputSameDT=on  OutDataTypeStr=Inherit: Same as first input
  Unit Delay1 : UnitDelay  SampleTime=Ts
  Unit Delay3 : UnitDelay  InitialCondition=Vc_Initial  SampleTime=Ts
  Unit Delay4 : UnitDelay  InitialCondition=Vc_Initial  SampleTime=Ts
  Vp : powerlib/Electrical Sources/Controlled Voltage Source  Initialize=off  Source_Type=AC  Amplitude=0  Phase=0  Frequency=0  Measurements=None
      settings: SourceProductName=Simscape Electrical
  Vp1 : powerlib/Electrical Sources/Controlled Voltage Source  Initialize=off  Source_Type=AC  Amplitude=0  Phase=0  Frequency=0  Measurements=None
      settings: SourceProductName=Simscape Electrical
  1 : PMIOPort  Side=Left
  2 : PMIOPort  Port=2  Side=Left
  Vc : Outport
  wires:
  N/1 -> Saturation1/1
  [Imod] -> Mux/1
  Unit Delay3/1 -> Sum2/2
  Unit Delay4/1 -> Unit Delay3/1, Gain2/1
  Gain2/1 -> Sum2/1
  Gain/1 -> Discrete-Time Integrator/1
  Discrete-Time Integrator/1 -> Unit Delay4/1
  Mux/1 -> Unit Delay1/1
  Product2/1 -> Demux/1
  Demux/1 -> [Vin]
  Demux/2 -> [Vbl]
  [Vin] -> Vp/1
  Current Measurement1/1 -> [Imod]
  Current Measurement2/1 -> [Icap]
  [Vbl] -> Vp1/1
  [Icap] -> Mux/2
  Unit Delay1/1 -> Product1/2
  Saturation1/1 -> Product1/1, Product2/1
  Product1/1 -> Sum1/1
  Sum2/1 -> Product2/2, Vc/1
  Sum1/1 -> Gain/1
  connections:
  1/RConn1 -- Vp/RConn1
  Vp/LConn1 -- Current Measurement1/LConn1
  Current Measurement1/RConn1 -- Dp/LConn1 -- Dp2/RConn1
  Current Measurement2/LConn1 -- Dp/RConn1
  Vp1/RConn1 -- Current Measurement2/RConn1
  Vp1/LConn1 -- 2/RConn1 -- Dp2/LConn1

== system clearing_faulted_segment_travelling_Wave/MMC Converter4/Half-Bridge MMC Ap1/HalfBridgeMMC_Agt_Discrete ==
  N : Inport  PortDimensions=2
  Current Measurement1 : powerlib/Measurements/Current Measurement  PhasorSimulation=off  OutputType=Complex  PSBequivalent=0
      settings: SourceProductName=Simscape Electrical
  Current Measurement2 : powerlib/Measurements/Current Measurement  PhasorSimulation=off  OutputType=Complex  PSBequivalent=0
      settings: SourceProductName=Simscape Electrical
  Demux : Demux  Outputs=2
  Discrete-Time Integrator : DiscreteIntegrator  IntegratorMethod=Integration: Trapezoidal  gainval=1  InitialCondition=Vc_Initial  SampleTime=Ts  UpperSaturationLimit=5000  LowerSaturationLimit=500  ICPrevOutput=DiscIntNeverNeededParam  ICPrevScaledInput=DiscIntNeverNeededParam
  Dp : powerlib/Power Electronics/Diode  Ron=Ron_Diode  Lon=0  Vf=Vf_Diode  IC=0  UseSnubber=off  Rs=Rs_Diode  Cs=Cs_Diode  Measurements=off
      settings: SourceProductName=Simscape Electrical
  Dp2 : powerlib/Power Electronics/Diode  Ron=Ron_Diode  Lon=0  Vf=Vf_Diode  IC=0  UseSnubber=off  Rs=Rs_Diode  Cs=Cs_Diode  Measurements=off
      settings: SourceProductName=Simscape Electrical
  Gain : Gain  Gain=1/(C*n)
  Gain2 : Gain  Gain=2
  Mux : Mux  Inputs=2
  Product1 : Product
  Product2 : Product
  Saturation1 : Saturate  UpperLimit=n  LowerLimit=0
  Sum1 : Sum  Inputs=1  SaturateOnIntegerOverflow=on  InputSameDT=on  OutDataTypeStr=Inherit: Same as first input
  Sum2 : Sum  Inputs=+-  SaturateOnIntegerOverflow=on  InputSameDT=on  OutDataTypeStr=Inherit: Same as first input
  Unit Delay1 : UnitDelay  SampleTime=Ts
  Unit Delay3 : UnitDelay  InitialCondition=Vc_Initial  SampleTime=Ts
  Unit Delay4 : UnitDelay  InitialCondition=Vc_Initial  SampleTime=Ts
  Vp : powerlib/Electrical Sources/Controlled Voltage Source  Initialize=off  Source_Type=AC  Amplitude=0  Phase=0  Frequency=0  Measurements=None
      settings: SourceProductName=Simscape Electrical
  Vp1 : powerlib/Electrical Sources/Controlled Voltage Source  Initialize=off  Source_Type=AC  Amplitude=0  Phase=0  Frequency=0  Measurements=None
      settings: SourceProductName=Simscape Electrical
  1 : PMIOPort  Side=Left
  2 : PMIOPort  Port=2  Side=Left
  Vc : Outport
  wires:
  N/1 -> Saturation1/1
  [Imod] -> Mux/1
  Unit Delay3/1 -> Sum2/2
  Unit Delay4/1 -> Unit Delay3/1, Gain2/1
  Gain2/1 -> Sum2/1
  Gain/1 -> Discrete-Time Integrator/1
  Discrete-Time Integrator/1 -> Unit Delay4/1
  Mux/1 -> Unit Delay1/1
  Product2/1 -> Demux/1
  Demux/1 -> [Vin]
  Demux/2 -> [Vbl]
  [Vin] -> Vp/1
  Current Measurement1/1 -> [Imod]
  Current Measurement2/1 -> [Icap]
  [Vbl] -> Vp1/1
  [Icap] -> Mux/2
  Unit Delay1/1 -> Product1/2
  Saturation1/1 -> Product1/1, Product2/1
  Product1/1 -> Sum1/1
  Sum2/1 -> Product2/2, Vc/1
  Sum1/1 -> Gain/1
  connections:
  1/RConn1 -- Vp/RConn1
  Vp/LConn1 -- Current Measurement1/LConn1
  Current Measurement1/RConn1 -- Dp/LConn1 -- Dp2/RConn1
  Current Measurement2/LConn1 -- Dp/RConn1
  Vp1/RConn1 -- Current Measurement2/RConn1
  Vp1/LConn1 -- 2/RConn1 -- Dp2/LConn1

== system clearing_faulted_segment_travelling_Wave/MMC Converter4/Half-Bridge MMC Ap2/HalfBridgeMMC_Agt_Discrete ==
  N : Inport  PortDimensions=2
  Current Measurement1 : powerlib/Measurements/Current Measurement  PhasorSimulation=off  OutputType=Complex  PSBequivalent=0
      settings: SourceProductName=Simscape Electrical
  Current Measurement2 : powerlib/Measurements/Current Measurement  PhasorSimulation=off  OutputType=Complex  PSBequivalent=0
      settings: SourceProductName=Simscape Electrical
  Demux : Demux  Outputs=2
  Discrete-Time Integrator : DiscreteIntegrator  IntegratorMethod=Integration: Trapezoidal  gainval=1  InitialCondition=Vc_Initial  SampleTime=Ts  UpperSaturationLimit=5000  LowerSaturationLimit=500  ICPrevOutput=DiscIntNeverNeededParam  ICPrevScaledInput=DiscIntNeverNeededParam
  Dp : powerlib/Power Electronics/Diode  Ron=Ron_Diode  Lon=0  Vf=Vf_Diode  IC=0  UseSnubber=off  Rs=Rs_Diode  Cs=Cs_Diode  Measurements=off
      settings: SourceProductName=Simscape Electrical
  Dp2 : powerlib/Power Electronics/Diode  Ron=Ron_Diode  Lon=0  Vf=Vf_Diode  IC=0  UseSnubber=off  Rs=Rs_Diode  Cs=Cs_Diode  Measurements=off
      settings: SourceProductName=Simscape Electrical
  Gain : Gain  Gain=1/(C*n)
  Gain2 : Gain  Gain=2
  Mux : Mux  Inputs=2
  Product1 : Product
  Product2 : Product
  Saturation1 : Saturate  UpperLimit=n  LowerLimit=0
  Sum1 : Sum  Inputs=1  SaturateOnIntegerOverflow=on  InputSameDT=on  OutDataTypeStr=Inherit: Same as first input
  Sum2 : Sum  Inputs=+-  SaturateOnIntegerOverflow=on  InputSameDT=on  OutDataTypeStr=Inherit: Same as first input
  Unit Delay1 : UnitDelay  SampleTime=Ts
  Unit Delay3 : UnitDelay  InitialCondition=Vc_Initial  SampleTime=Ts
  Unit Delay4 : UnitDelay  InitialCondition=Vc_Initial  SampleTime=Ts
  Vp : powerlib/Electrical Sources/Controlled Voltage Source  Initialize=off  Source_Type=AC  Amplitude=0  Phase=0  Frequency=0  Measurements=None
      settings: SourceProductName=Simscape Electrical
  Vp1 : powerlib/Electrical Sources/Controlled Voltage Source  Initialize=off  Source_Type=AC  Amplitude=0  Phase=0  Frequency=0  Measurements=None
      settings: SourceProductName=Simscape Electrical
  1 : PMIOPort  Side=Left
  2 : PMIOPort  Port=2  Side=Left
  Vc : Outport
  wires:
  Sum1/1 -> Gain/1
  Sum2/1 -> Vc/1, Product2/2
  Product1/1 -> Sum1/1
  Saturation1/1 -> Product2/1, Product1/1
  Unit Delay1/1 -> Product1/2
  [Icap] -> Mux/2
  [Vbl] -> Vp1/1
  Current Measurement2/1 -> [Icap]
  Current Measurement1/1 -> [Imod]
  [Vin] -> Vp/1
  Demux/2 -> [Vbl]
  Demux/1 -> [Vin]
  Product2/1 -> Demux/1
  Mux/1 -> Unit Delay1/1
  Discrete-Time Integrator/1 -> Unit Delay4/1
  Gain/1 -> Discrete-Time Integrator/1
  Gain2/1 -> Sum2/1
  Unit Delay4/1 -> Gain2/1, Unit Delay3/1
  Unit Delay3/1 -> Sum2/2
  [Imod] -> Mux/1
  N/1 -> Saturation1/1
  connections:
  Dp2/LConn1 -- 2/RConn1 -- Vp1/LConn1
  Vp1/RConn1 -- Current Measurement2/RConn1
  Current Measurement2/LConn1 -- Dp/RConn1
  Dp2/RConn1 -- Dp/LConn1 -- Current Measurement1/RConn1
  Vp/LConn1 -- Current Measurement1/LConn1
  1/RConn1 -- Vp/RConn1

== system clearing_faulted_segment_travelling_Wave/MMC Converter4/Half-Bridge MMC Ap3/HalfBridgeMMC_Agt_Discrete ==
  N : Inport  PortDimensions=2
  Current Measurement1 : powerlib/Measurements/Current Measurement  PhasorSimulation=off  OutputType=Complex  PSBequivalent=0
      settings: SourceProductName=Simscape Electrical
  Current Measurement2 : powerlib/Measurements/Current Measurement  PhasorSimulation=off  OutputType=Complex  PSBequivalent=0
      settings: SourceProductName=Simscape Electrical
  Demux : Demux  Outputs=2
  Discrete-Time Integrator : DiscreteIntegrator  IntegratorMethod=Integration: Trapezoidal  gainval=1  InitialCondition=Vc_Initial  SampleTime=Ts  UpperSaturationLimit=5000  LowerSaturationLimit=500  ICPrevOutput=DiscIntNeverNeededParam  ICPrevScaledInput=DiscIntNeverNeededParam
  Dp : powerlib/Power Electronics/Diode  Ron=Ron_Diode  Lon=0  Vf=Vf_Diode  IC=0  UseSnubber=off  Rs=Rs_Diode  Cs=Cs_Diode  Measurements=off
      settings: SourceProductName=Simscape Electrical
  Dp2 : powerlib/Power Electronics/Diode  Ron=Ron_Diode  Lon=0  Vf=Vf_Diode  IC=0  UseSnubber=off  Rs=Rs_Diode  Cs=Cs_Diode  Measurements=off
      settings: SourceProductName=Simscape Electrical
  Gain : Gain  Gain=1/(C*n)
  Gain2 : Gain  Gain=2
  Mux : Mux  Inputs=2
  Product1 : Product
  Product2 : Product
  Saturation1 : Saturate  UpperLimit=n  LowerLimit=0
  Sum1 : Sum  Inputs=1  SaturateOnIntegerOverflow=on  InputSameDT=on  OutDataTypeStr=Inherit: Same as first input
  Sum2 : Sum  Inputs=+-  SaturateOnIntegerOverflow=on  InputSameDT=on  OutDataTypeStr=Inherit: Same as first input
  Unit Delay1 : UnitDelay  SampleTime=Ts
  Unit Delay3 : UnitDelay  InitialCondition=Vc_Initial  SampleTime=Ts
  Unit Delay4 : UnitDelay  InitialCondition=Vc_Initial  SampleTime=Ts
  Vp : powerlib/Electrical Sources/Controlled Voltage Source  Initialize=off  Source_Type=AC  Amplitude=0  Phase=0  Frequency=0  Measurements=None
      settings: SourceProductName=Simscape Electrical
  Vp1 : powerlib/Electrical Sources/Controlled Voltage Source  Initialize=off  Source_Type=AC  Amplitude=0  Phase=0  Frequency=0  Measurements=None
      settings: SourceProductName=Simscape Electrical
  1 : PMIOPort  Side=Left
  2 : PMIOPort  Port=2  Side=Left
  Vc : Outport
  wires:
  Sum1/1 -> Gain/1
  Sum2/1 -> Vc/1, Product2/2
  Product1/1 -> Sum1/1
  Saturation1/1 -> Product2/1, Product1/1
  Unit Delay1/1 -> Product1/2
  [Icap] -> Mux/2
  [Vbl] -> Vp1/1
  Current Measurement2/1 -> [Icap]
  Current Measurement1/1 -> [Imod]
  [Vin] -> Vp/1
  Demux/2 -> [Vbl]
  Demux/1 -> [Vin]
  Product2/1 -> Demux/1
  Mux/1 -> Unit Delay1/1
  Discrete-Time Integrator/1 -> Unit Delay4/1
  Gain/1 -> Discrete-Time Integrator/1
  Gain2/1 -> Sum2/1
  Unit Delay4/1 -> Gain2/1, Unit Delay3/1
  Unit Delay3/1 -> Sum2/2
  [Imod] -> Mux/1
  N/1 -> Saturation1/1
  connections:
  Dp2/LConn1 -- 2/RConn1 -- Vp1/LConn1
  Vp1/RConn1 -- Current Measurement2/RConn1
  Current Measurement2/LConn1 -- Dp/RConn1
  Dp2/RConn1 -- Dp/LConn1 -- Current Measurement1/RConn1
  Vp/LConn1 -- Current Measurement1/LConn1
  1/RConn1 -- Vp/RConn1

== system clearing_faulted_segment_travelling_Wave/MMC Converter4/Half-Bridge MMC Ap4/HalfBridgeMMC_Agt_Discrete ==
  N : Inport  PortDimensions=2
  Current Measurement1 : powerlib/Measurements/Current Measurement  PhasorSimulation=off  OutputType=Complex  PSBequivalent=0
      settings: SourceProductName=Simscape Electrical
  Current Measurement2 : powerlib/Measurements/Current Measurement  PhasorSimulation=off  OutputType=Complex  PSBequivalent=0
      settings: SourceProductName=Simscape Electrical
  Demux : Demux  Outputs=2
  Discrete-Time Integrator : DiscreteIntegrator  IntegratorMethod=Integration: Trapezoidal  gainval=1  InitialCondition=Vc_Initial  SampleTime=Ts  UpperSaturationLimit=5000  LowerSaturationLimit=500  ICPrevOutput=DiscIntNeverNeededParam  ICPrevScaledInput=DiscIntNeverNeededParam
  Dp : powerlib/Power Electronics/Diode  Ron=Ron_Diode  Lon=0  Vf=Vf_Diode  IC=0  UseSnubber=off  Rs=Rs_Diode  Cs=Cs_Diode  Measurements=off
      settings: SourceProductName=Simscape Electrical
  Dp2 : powerlib/Power Electronics/Diode  Ron=Ron_Diode  Lon=0  Vf=Vf_Diode  IC=0  UseSnubber=off  Rs=Rs_Diode  Cs=Cs_Diode  Measurements=off
      settings: SourceProductName=Simscape Electrical
  Gain : Gain  Gain=1/(C*n)
  Gain2 : Gain  Gain=2
  Mux : Mux  Inputs=2
  Product1 : Product
  Product2 : Product
  Saturation1 : Saturate  UpperLimit=n  LowerLimit=0
  Sum1 : Sum  Inputs=1  SaturateOnIntegerOverflow=on  InputSameDT=on  OutDataTypeStr=Inherit: Same as first input
  Sum2 : Sum  Inputs=+-  SaturateOnIntegerOverflow=on  InputSameDT=on  OutDataTypeStr=Inherit: Same as first input
  Unit Delay1 : UnitDelay  SampleTime=Ts
  Unit Delay3 : UnitDelay  InitialCondition=Vc_Initial  SampleTime=Ts
  Unit Delay4 : UnitDelay  InitialCondition=Vc_Initial  SampleTime=Ts
  Vp : powerlib/Electrical Sources/Controlled Voltage Source  Initialize=off  Source_Type=AC  Amplitude=0  Phase=0  Frequency=0  Measurements=None
      settings: SourceProductName=Simscape Electrical
  Vp1 : powerlib/Electrical Sources/Controlled Voltage Source  Initialize=off  Source_Type=AC  Amplitude=0  Phase=0  Frequency=0  Measurements=None
      settings: SourceProductName=Simscape Electrical
  1 : PMIOPort  Side=Left
  2 : PMIOPort  Port=2  Side=Left
  Vc : Outport
  wires:
  N/1 -> Saturation1/1
  [Imod] -> Mux/1
  Unit Delay3/1 -> Sum2/2
  Unit Delay4/1 -> Unit Delay3/1, Gain2/1
  Gain2/1 -> Sum2/1
  Gain/1 -> Discrete-Time Integrator/1
  Discrete-Time Integrator/1 -> Unit Delay4/1
  Mux/1 -> Unit Delay1/1
  Product2/1 -> Demux/1
  Demux/1 -> [Vin]
  Demux/2 -> [Vbl]
  [Vin] -> Vp/1
  Current Measurement1/1 -> [Imod]
  Current Measurement2/1 -> [Icap]
  [Vbl] -> Vp1/1
  [Icap] -> Mux/2
  Unit Delay1/1 -> Product1/2
  Saturation1/1 -> Product1/1, Product2/1
  Product1/1 -> Sum1/1
  Sum2/1 -> Product2/2, Vc/1
  Sum1/1 -> Gain/1
  connections:
  1/RConn1 -- Vp/RConn1
  Vp/LConn1 -- Current Measurement1/LConn1
  Current Measurement1/RConn1 -- Dp/LConn1 -- Dp2/RConn1
  Current Measurement2/LConn1 -- Dp/RConn1
  Vp1/RConn1 -- Current Measurement2/RConn1
  Vp1/LConn1 -- 2/RConn1 -- Dp2/LConn1
